simulink model "cart_pendulum_coupled_model"  (R2015b)
settings: Solver=ode23  StartTime=0.0  StopTime=tsimu  RelTol=1e-3
values from neighbouring files (symbols this model uses):
  A = 0.18/2    (= 0.09)    [simulation_coupled_model.m]
  B = 20    [simulation_coupled_model.m]
  cart_pos_0 = -A    (= -0.09)    [simulation_coupled_model.m]
  cart_vel_0 = 0.    (= 0)    [simulation_coupled_model.m]
  d = 0.45    [simulation_coupled_model.m]
  f = 0.64    [simulation_coupled_model.m]
  g = 9.81    [simulation_coupled_model.m]
  K = 120    [simulation_coupled_model.m]
  mc = 2.4    [simulation_coupled_model.m]
  mp = 0.6    [simulation_coupled_model.m]
  omega_0 = 0.    (= 0)    [simulation_coupled_model.m]
  theta_0 = 0.    (= 0)    [simulation_coupled_model.m]
settings Model: Creator=pauline  LastModifiedBy=pauline
settings SolverCC: ZeroCrossAlgorithm=Adaptive  AlgebraicLoopSolver=LineSearch

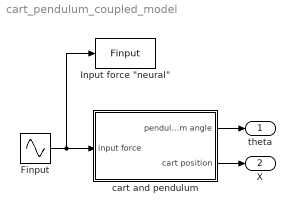
== system cart_pendulum_coupled_model ==
  Finput : Sin  Amplitude=A*(mp+mc)*(2*pi*f)*(2*pi*f)  Frequency=2*pi*f  Phase=pi/2  SampleTime=0
  "Input force \"neural\"" : ToWorkspace  VariableName=Finput  SaveFormat=Timeseries  SampleTime=-1
  cart and pendulum : Subsystem
  theta : Outport
  X : Outport  Port=2
  wires:
  cart and pendulum/1(pendulum angle) -> theta/1
  Finput/1 -> cart and pendulum/1(input force), "Input force \"neural\""/1
  cart and pendulum/2(cart position) -> X/1

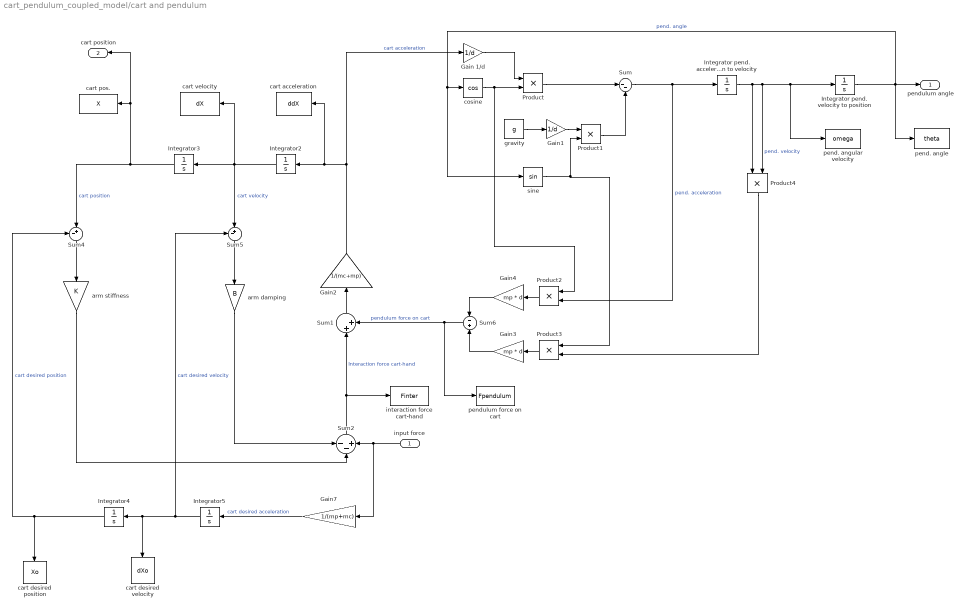
== system cart_pendulum_coupled_model/cart and pendulum ==
  input force : Inport
  Gain 1/d : Gain  Gain=1/d
  Gain1 : Gain  Gain=1/d
  Gain2 : Gain  Gain=1/(mc+mp)
  Gain3 : Gain  Gain=mp * d
  Gain4 : Gain  Gain=mp * d
  Gain7 : Gain  Gain=1/(mp+mc)
  Integrator pend. acceleration to velocity : Integrator  InitialCondition=omega_0
  Integrator pend. velocity to position : Integrator  InitialCondition=theta_0
  Integrator2 : Integrator  InitialCondition=cart_vel_0
  Integrator3 : Integrator  InitialCondition=cart_pos_0
  Integrator4 : Integrator  InitialCondition=cart_pos_0
  Integrator5 : Integrator  InitialCondition=cart_vel_0
  Product{,1..4} (5 alike) : Product
  Sum : Sum  Inputs=|--
  Sum1 : Sum  Inputs=|++
  Sum2 : Sum  Inputs=--+
  Sum4 : Sum  Inputs=-+|
  Sum5 : Sum  Inputs=-+|
  Sum6 : Sum  Inputs=-|+
  arm damping : Gain  Gain=B
  arm stiffness : Gain  Gain=K
  cart acceleration : ToWorkspace  VariableName=ddX  SaveFormat=Timeseries  SampleTime=-1
  "cart desired position " : ToWorkspace  VariableName=Xo  SaveFormat=Timeseries  SampleTime=-1
  cart desired velocity : ToWorkspace  VariableName=dXo  SaveFormat=Timeseries  SampleTime=-1
  cart pos. : ToWorkspace  VariableName=X  SaveFormat=Timeseries  SampleTime=-1
  cart velocity : ToWorkspace  VariableName=dX  SaveFormat=Timeseries  SampleTime=-1
  cosine : Trigonometry  Operator=cos
  gravity : Constant  Value=g
  interaction force cart-hand : ToWorkspace  VariableName=Finter  SaveFormat=Timeseries  SampleTime=-1
  pend. angle : ToWorkspace  VariableName=theta  SaveFormat=Timeseries  SampleTime=-1
  pend. angular velocity : ToWorkspace  VariableName=omega  SaveFormat=Timeseries  SampleTime=-1
  pendulum force on cart : ToWorkspace  VariableName=Fpendulum  SaveFormat=Timeseries  SampleTime=-1
  sine : Trigonometry
  pendulum angle : Outport
  cart position : Outport  Port=2
  wires:
  Product/1 -> Sum/1
  Product1/1 -> Sum/2
  cosine/1 -> Product/2, Product2/1
  Gain 1/d/1 -> Product/1
  Gain1/1 -> Product1/1
  sine/1 -> Product3/1, Product1/2
  gravity/1 -> Gain1/1
  Product2/1 -> Gain4/1
  Product3/1 -> Gain3/1
  Sum/1 -> Product2/2, Integrator pend. acceleration to velocity/1  "pend. acceleration"
  Integrator pend. acceleration to velocity/1 -> Product4/2, Integrator pend. velocity to position/1, pend. angular velocity/1, Product4/1  "pend. velocity"
  Product4/1 -> Product3/2
  Integrator pend. velocity to position/1 -> sine/1, cosine/1, pendulum angle/1, pend. angle/1  "pend. angle"
  Integrator3/1 -> cart position/1, cart pos./1, Sum4/2  "cart position"
  Sum4/1 -> arm stiffness/1
  Sum5/1 -> arm damping/1
  Gain7/1 -> Integrator5/1  "cart desired acceleration"
  Integrator5/1 -> Sum5/1, Integrator4/1, cart desired velocity/1  "cart desired velocity"
  Integrator4/1 -> Sum4/1, "cart desired position "/1  "cart desired position"
  Sum6/1 -> Sum1/2, pendulum force on cart/1  "pendulum force on cart"
  Gain4/1 -> Sum6/1
  Gain3/1 -> Sum6/2
  Sum2/1 -> Sum1/1, interaction force cart-hand/1  "Interaction force cart-hand"
  input force/1 -> Gain7/1, Sum2/3
  Sum1/1 -> Gain2/1
  Gain2/1 -> Gain 1/d/1, cart acceleration/1, Integrator2/1  "cart acceleration"
  Integrator2/1 -> Sum5/2, cart velocity/1, Integrator3/1  "cart velocity"
  arm damping/1 -> Sum2/1
  arm stiffness/1 -> Sum2/2
